simulink model "Ejercicio2correcto"  (R2012b)
settings: Solver=ode45  StartTime=0.0  StopTime=10.0  RelTol=1e-3
values from neighbouring files (symbols this model uses):
  a = [0 -1;-1 0]    [Ejercicio2.m]
  b = [0;1]    [Ejercicio2.m]
  c = [1,0]    [Ejercicio2.m]
  h = h'    [Ejercicio2.m]
  hdis = hdis'    [Ejercicio2.m]
  ki = kt(1,3)    [Ejercicio2.m]
  kidis = ktdis(1,3)    [Ejercicio2.m]
  kp = kt(1,1:2)    [Ejercicio2.m]
  kpdis = ktdis(1,1:2)    [Ejercicio2.m]
undefined symbols (not defined in the file or in its folder): adis, bdis, cdis
settings Model: Creator=tp.aulas3  LastModifiedBy=carlos_mar.paredes
settings DataIOCC: SignalLoggingSaveFormat=ModelDataLogs
settings OptimizationCC: ExpressionDepthLimit=128
settings DebuggingCC: MultiTaskDSMMsg=warning  MultiTaskCondExecSysMsg=none  StrictBusMsg=None
settings RTWCC: IncludeERTFirstTime=on
settings CodeAppCC: CustomSymbolStrType=$N$R$M_T  InternalIdentifier=Shortened

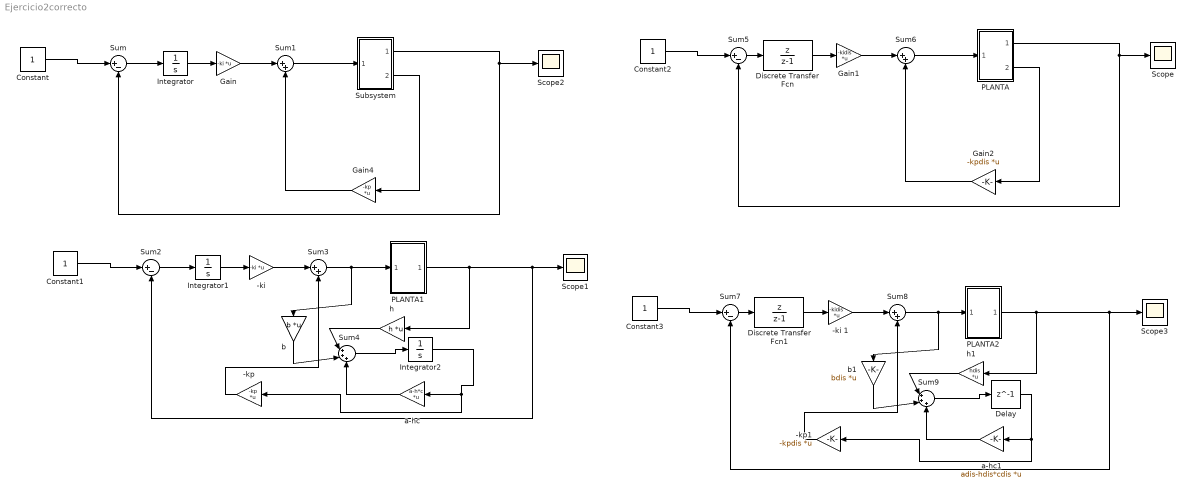
== system Ejercicio2correcto ==
  "-ki " : Gain  Gain=-ki  Multiplication=Matrix(K*u) (u vector)
  -ki 1 : Gain  Gain=-kidis  Multiplication=Matrix(K*u) (u vector)  SampleTime=0.1
  -kp : Gain  Gain=-kp  Multiplication=Matrix(K*u) (u vector)
  -kp1 : Gain  Gain=-kpdis  Multiplication=Matrix(K*u) (u vector)  SampleTime=0.1
  Constant : Constant
  Constant1 : Constant
  Constant2 : Constant  SampleTime=0.1
  Constant3 : Constant  SampleTime=0.1
  Delay : Delay  DelayLength=1  SampleTime=0.1
  Discrete Transfer Fcn : DiscreteTransferFcn  Numerator=[1 0]  Denominator=[1 -1]  SampleTime=0.1
  Discrete Transfer Fcn1 : DiscreteTransferFcn  Numerator=[1 0]  Denominator=[1 -1]  SampleTime=0.1
  Gain : Gain  Gain=-ki  Multiplication=Matrix(K*u) (u vector)
  Gain1 : Gain  Gain=-kidis  Multiplication=Matrix(K*u) (u vector)  SampleTime=0.1
  Gain2 : Gain  Gain=-kpdis  Multiplication=Matrix(K*u) (u vector)  SampleTime=0.1
  Gain4 : Gain  Gain=-kp  Multiplication=Matrix(K*u) (u vector)
  Integrator : Integrator
  Integrator1 : Integrator
  Integrator2 : Integrator
  PLANTA : Subsystem
  PLANTA1 : Subsystem
  PLANTA2 : Subsystem
  Scope{,1..3} (4 alike) : Scope
      Scope settings: SaveName=ScopeData2
      Scope3 settings: SaveName=ScopeData3
  Subsystem : Subsystem
  Sum : Sum  Inputs=|+-
  Sum1 : Sum  Inputs=|++
  Sum2 : Sum  Inputs=|+-
  Sum3 : Sum  Inputs=|++
  Sum4 : Sum  Inputs=|+++
  Sum5 : Sum  Inputs=|+-  SampleTime=0.1
  Sum6 : Sum  Inputs=|++  SampleTime=0.1
  Sum7 : Sum  Inputs=|+-  SampleTime=0.1
  Sum8 : Sum  Inputs=|++  SampleTime=0.1
  Sum9 : Sum  Inputs=|+++  SampleTime=0.1
  a-hc : Gain  Gain=a-h*c  Multiplication=Matrix(K*u) (u vector)
  a-hc1 : Gain  Gain=adis-hdis*cdis  Multiplication=Matrix(K*u) (u vector)  SampleTime=0.1
  b : Gain  Gain=b  Multiplication=Matrix(K*u) (u vector)
  b1 : Gain  Gain=bdis  Multiplication=Matrix(K*u) (u vector)  SampleTime=0.1
  h : Gain  Gain=h  Multiplication=Matrix(K*u) (u vector)
  h1 : Gain  Gain=hdis  Multiplication=Matrix(K*u) (u vector)  SampleTime=0.1
  wires:
  Sum/1 -> Integrator/1
  Integrator/1 -> Gain/1
  Gain/1 -> Sum1/1
  Gain4/1 -> Sum1/2
  Constant/1 -> Sum/1
  Subsystem/1(Out1) -> Scope2/1, Sum/2
  Sum1/1 -> Subsystem/1(In1)
  Subsystem/2(Out2) -> Gain4/1
  Sum2/1 -> Integrator1/1
  Integrator1/1 -> "-ki "/1
  "-ki "/1 -> Sum3/1
  Constant1/1 -> Sum2/1
  PLANTA1/1(Out1) -> h/1, Scope1/1, Sum2/2
  Sum3/1 -> b/1, PLANTA1/1(In1)
  h/1 -> Sum4/1
  b/1 -> Sum4/2
  Sum4/1 -> Integrator2/1
  Integrator2/1 -> -kp/1, a-hc/1
  a-hc/1 -> Sum4/3
  -kp/1 -> Sum3/2
  Gain1/1 -> Sum6/1
  Gain2/1 -> Sum6/2
  Constant2/1 -> Sum5/1
  PLANTA/1(Out1) -> Sum5/2, Scope/1
  Sum6/1 -> PLANTA/1(In1)
  PLANTA/2(Out2) -> Gain2/1
  -ki 1/1 -> Sum8/1
  Constant3/1 -> Sum7/1
  Sum8/1 -> PLANTA2/1(In1), b1/1
  h1/1 -> Sum9/1
  b1/1 -> Sum9/2
  a-hc1/1 -> Sum9/3
  -kp1/1 -> Sum8/2
  Sum5/1 -> Discrete Transfer Fcn/1
  Discrete Transfer Fcn/1 -> Gain1/1
  PLANTA2/1(Out1) -> h1/1, Sum7/2, Scope3/1
  Sum7/1 -> Discrete Transfer Fcn1/1
  Discrete Transfer Fcn1/1 -> -ki 1/1
  Sum9/1 -> Delay/1
  Delay/1 -> -kp1/1, a-hc1/1

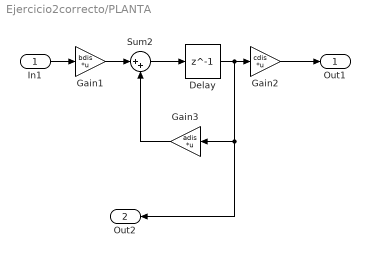
== system Ejercicio2correcto/PLANTA ==
  In1 : Inport
  Delay : Delay  DelayLength=1
  Gain1 : Gain  Gain=bdis  Multiplication=Matrix(K*u) (u vector)  SampleTime=0.1
  Gain2 : Gain  Gain=cdis  Multiplication=Matrix(K*u) (u vector)  SampleTime=0.1
  Gain3 : Gain  Gain=adis  Multiplication=Matrix(K*u) (u vector)  SampleTime=0.1
  Sum2 : Sum  Inputs=|++  SampleTime=0.1
  Out1 : Outport
  Out2 : Outport  Port=2
  wires:
  Delay/1 -> Out2/1, Gain3/1, Gain2/1
  In1/1 -> Gain1/1
  Gain1/1 -> Sum2/1
  Gain3/1 -> Sum2/2
  Gain2/1 -> Out1/1
  Sum2/1 -> Delay/1

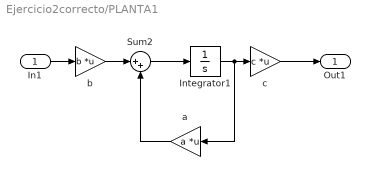
== system Ejercicio2correcto/PLANTA1 ==
  In1 : Inport
  Integrator1 : Integrator
  Sum2 : Sum  Inputs=|++
  a : Gain  Gain=a  Multiplication=Matrix(K*u) (u vector)
  b : Gain  Gain=b  Multiplication=Matrix(K*u) (u vector)
  c : Gain  Gain=c  Multiplication=Matrix(K*u) (u vector)
  Out1 : Outport
  wires:
  Sum2/1 -> Integrator1/1
  c/1 -> Out1/1
  a/1 -> Sum2/2
  b/1 -> Sum2/1
  In1/1 -> b/1
  Integrator1/1 -> c/1, a/1

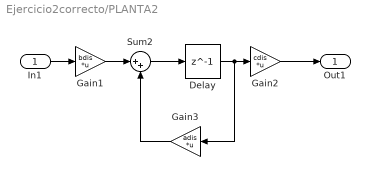
== system Ejercicio2correcto/PLANTA2 ==
  In1 : Inport
  Delay : Delay  DelayLength=1
  Gain1 : Gain  Gain=bdis  Multiplication=Matrix(K*u) (u vector)  SampleTime=0.1
  Gain2 : Gain  Gain=cdis  Multiplication=Matrix(K*u) (u vector)  SampleTime=0.1
  Gain3 : Gain  Gain=adis  Multiplication=Matrix(K*u) (u vector)  SampleTime=0.1
  Sum2 : Sum  Inputs=|++  SampleTime=0.1
  Out1 : Outport
  wires:
  Delay/1 -> Gain3/1, Gain2/1
  In1/1 -> Gain1/1
  Gain1/1 -> Sum2/1
  Gain3/1 -> Sum2/2
  Gain2/1 -> Out1/1
  Sum2/1 -> Delay/1

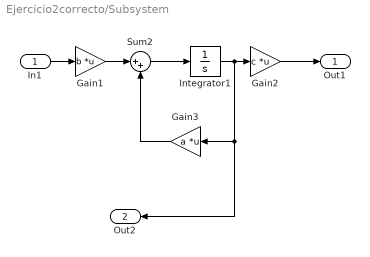
== system Ejercicio2correcto/Subsystem ==
  In1 : Inport
  Gain1 : Gain  Gain=b  Multiplication=Matrix(K*u) (u vector)
  Gain2 : Gain  Gain=c  Multiplication=Matrix(K*u) (u vector)
  Gain3 : Gain  Gain=a  Multiplication=Matrix(K*u) (u vector)
  Integrator1 : Integrator
  Sum2 : Sum  Inputs=|++
  Out1 : Outport
  Out2 : Outport  Port=2
  wires:
  Integrator1/1 -> Out2/1, Gain3/1, Gain2/1
  In1/1 -> Gain1/1
  Gain1/1 -> Sum2/1
  Gain3/1 -> Sum2/2
  Gain2/1 -> Out1/1
  Sum2/1 -> Integrator1/1
